simulink model "UnitTestWellClearMetrics"  (R2018b)
settings: Solver=FixedStepDiscrete  StartTime=0.0  StopTime=t_stop  FixedStep=1  RelTol=1e-3  EnableMultiTasking=on
libraries: WellClearMetricsBlock x1
settings Model: Creator=RA24876  LastModifiedBy=BI28030
settings DataIOCC: LimitDataPoints=on  SaveFormat=Array
settings OptimizationCC: ExpressionDepthLimit=2147483647  LifeSpan=inf
settings DebuggingCC: UnderspecifiedInitializationDetection=Classic  MergeDetectMultiDrivingBlocksExec=none  SolverPrmCheckMsg=warning  StateNameClashWarn=warning  SFUnexpectedBacktrackingDiag=warning  SFNoUnconditionalDefaultTransitionDiag=warning  SFExecutionAtInitializationDiag=none
settings HardwareCC: ProdBitPerPointer=32  ProdBitPerSizeT=32  ProdBitPerPtrDiffT=32  ProdLargestAtomicFloat=None  ProdIntDivRoundTo=Undefined  ProdEndianess=Unspecified  ProdWordSize=32  ProdHWDeviceType=32-bit Generic
settings ModelReferenceCC: PropagateSignalLabelsOutOfModel=off
settings SFSimCC: SimUseLocalCustomCode=off
settings RTWCC: RTWUseLocalCustomCode=off
settings CodeAppCC: StateflowObjectComments=on
settings GRTTargetCC: TargetLangStandard=C89/C90 (ANSI)  GeneratePreprocessorConditionals=Disable all
settings ConfigComp: CovMetricSettings=dw  CovHtmlReporting=on  CovSaveCumulativeToWorkspaceVar=on  CovSaveSingleToWorkspaceVar=on  CovExternalEMLEnable=off

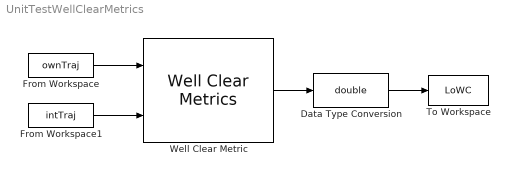
== system UnitTestWellClearMetrics ==
  Data Type Conversion : DataTypeConversion  OutDataTypeStr=double
  From Workspace : FromWorkspace  VariableName=ownTraj  SampleTime=0
  From Workspace1 : FromWorkspace  VariableName=intTraj  SampleTime=0
  To Workspace : ToWorkspace  VariableName=LoWC  SampleTime=-1
  Well Clear Metric : WellClearMetricsBlock/Well Clear Metrics  tauThreshold=35  hmdThreshold=4000  tauVThreshold=0  altThreshold=700  rngThreshold=4000
  wires:
  Well Clear Metric/1 -> Data Type Conversion/1
  Data Type Conversion/1 -> To Workspace/1
  From Workspace/1 -> Well Clear Metric/1
  From Workspace1/1 -> Well Clear Metric/2
